simulink model "innerlooptester"  (Simulink 8.7)
settings: Solver=ode45  StartTime=0.0  StopTime=40  RelTol=1e-9
settings Model: Creator=tommi  LastModifiedBy=tommi
settings DataIOCC: SignalLoggingSaveFormat=ModelDataLogs
settings OptimizationCC: ExpressionDepthLimit=2147483647
settings DebuggingCC: SolverPrmCheckMsg=warning  FcnCallInpInsideContextMsg=EnableAllAsWarning  StateNameClashWarn=warning

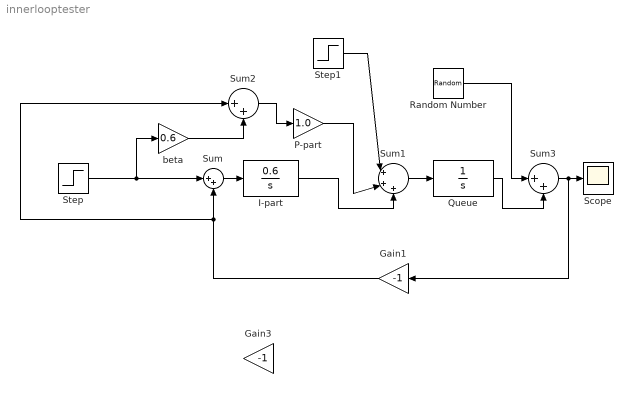
== system innerlooptester ==
  Gain1 : Gain  Gain=-1
  Gain3 : Gain  Gain=-1
  I-part : TransferFcn  Numerator=[0.6]  Denominator=[1 0]
  P-part : Gain  Gain=1.0
  Queue : TransferFcn  Denominator=[1 0]
  Random Number : RandomNumber  Variance=0
  Scope : Scope
  Step : Step  Time=0  SampleTime=0
  Step1 : Step  Time=20  After=-0.5  SampleTime=0
  Sum : Sum  Inputs=|++
  Sum1 : Sum  Inputs=|+++
  Sum2 : Sum  Inputs=|++
  Sum3 : Sum  Inputs=|++
  beta : Gain  Gain=0.6
  wires:
  Gain1/1 -> Sum/2, Sum2/1
  Sum/1 -> I-part/1
  Sum1/1 -> Queue/1
  Step1/1 -> Sum1/1
  Step/1 -> Sum/1, beta/1
  I-part/1 -> Sum1/3
  beta/1 -> Sum2/2
  Sum2/1 -> P-part/1
  P-part/1 -> Sum1/2
  Sum3/1 -> Gain1/1, Scope/1
  Random Number/1 -> Sum3/1
  Queue/1 -> Sum3/2
